simulink model "rx"  (R2019b)
settings: Solver=FixedStepDiscrete  StartTime=0.0  StopTime=inf  RelTol=1e-3
undefined symbols (not defined in the file): F, usb
libraries: plutoradiolib x1, commsink2 x1, zc706fmc234_lib x1
settings Model: Creator=tcollins  LastModifiedBy=bhisma
settings DataIOCC: ReturnWorkspaceOutputs=off
settings DebuggingCC: ArithmeticOperatorsInVariantConditions=warning
settings SFSimCC: SimUseLocalCustomCode=off  CustomCodeUndefinedFunction=UseInterfaceOnly
settings RTWCC: RTWUseLocalCustomCode=off

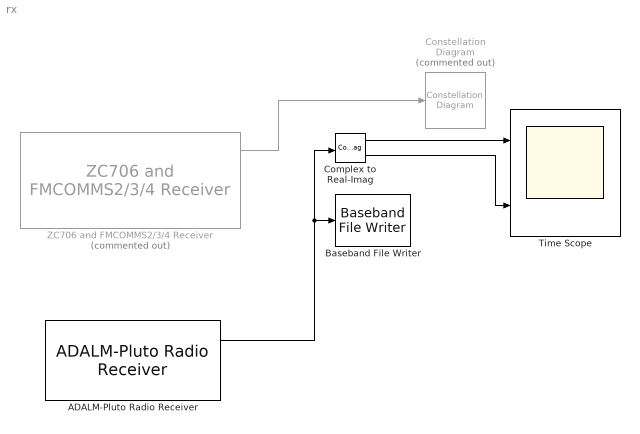
== system rx ==
  ADALM-Pluto Radio Receiver : plutoradiolib/ADALM-Pluto Radio Receiver  SourceLibraryInfo="This block requires <a href=\"http://www.mathworks.com/hardware-support/rtl-sdr.html\">Communications System Toolbox Support Package for RTL-SDR Radio</a>"  RadioID=usb:0  CenterFrequencySource=Dialog  CenterFrequency=2.4e9  GainSource=AGC Slow Attack  Gain=10  ChannelMapping=1  BasebandSampleRate=1e6  OutputDataType=int16  SamplesPerFrame=2^15  OverflowOutputPort=on  SimulateUsing=Interpreted execution  EnableQuadratureTracking=on  EnableRFDCTracking=on  EnableBasebandDCTracking=on
      settings: SourceProductName=Communications System Toolbox Support Package for ADALM-PLUTO Radio
  Baseband File Writer : commsink2/Baseband File Writer  Filename=untitled.bb  CenterFrequency=950e6  Metadata=struct()  NumSamplesToWrite=1e6  SimulateUsing=Code generation
      settings: SourceProductName=Communications Toolbox  SourceProductBaseCode=CM
  Complex to Real-Imag : ComplexToRealImag
  Constellation Diagram : ConstellationDiagram  Commented=on
  Time Scope : Scope  NumInputPorts=2
  ZC706 and FMCOMMS2/3/4 Receiver : zc706fmc234_lib/ZC706 and  FMCOMMS2//3//4  Receiver  Commented=on  IPAddress=192.168.3.2  CenterFrequencySource=Dialog  CenterFrequency=2.4e9  GainSource=AGC Slow Attack  Gain=1  ChannelMapping=1  BasebandSampleRate=20e6  EnableBurstMode=off  NumFramesInBurst=20  OutputDataType=int16  SamplesPerFrame=2^15  LostSamplesOutputPort=on  RSSIOutputPort=off  DMATimeoutValue=1  blockMode=Normal  SimulateUsing=Code generation  EnableQuadratureTracking=on  EnableRFDCTracking=on  EnableBasebandDCTracking=on  BypassUserLogic=on  ShowAdvancedProperties=on  ShowInternalProperties=off  subDeviceList=zynqReceiver  sdrExecutionMode=HW  dataUDPPort=-1  ctrlUDPPort=-1  SourceSelect=RF data  SourceConfiguration1=1023  FIRCoefficientSize=[128;128]  FIRCoefficients=[55 -54 42 -126 -123 -317 -399 -581 -646 -711 -634 -507 -263 -10 255 424 492 401 201 -84 -352 -540 -566 -423 -126 234 562 738 701 429 -5 -490 -866 -1007 -834 -372 266 891 1301 1334 936 178 -733 -1524 -1917 -1731 -944 274 1590 2585 2881 2255 741 -1344 -3435 -4850 -4942 -3285 197 5169 10923 16509 20932 23375 23375 20932 16509 10923 5169 197 -3285 -4942 -4850 -3435 -1344 741 2255 2881 2585 1590 274 -944 -1731 -1917 -1524 -733 178 936 1334 1301 891 266 -372 -834 -1007 -866 -490 -5 429 701 738 562 234 -126 -423 -566 -540 -352 -84 201 401 492 424 255 -10 -263 -507 -634 -711 -646 -581 -399 -317 -123 -126 42 -54 55;190 -88 329 -40 239 -99 -24 -349 -377 -611 -573 -604 -395 -229 66 239 394 350 227 -46 -300 -534 -593 -506 -221 137 512 737 765 526 103 -420 -852 -1069 -947 -512 156 841 1341 1450 1100 333 -638 -1531 -2028 -1922 -1152 115 1544 2677 3099 2535 997 -1205 -3479 -5095 -5345 -3750 -199 4965 11002 16895 21580 24172 24172 21580 16895 11002 4965 -199 -3750 -5345 -5095 -3479 -1205 997 2535 3099 2677 1544 115 -1152 -1922 -2028 -1531 -638 333 1100 1450 1341 841 156 -512 -947 -1069 -852 -420 103 526 765 737 512 137 -221 -506 -593 -534 -300 -46 227 350 394 239 66 -229 -395 -604 -573 -611 -377 -349 -24 -99 239 -40 329 -88 190]  FIRGain=[0;-12]  FIRDecimInterpFactor=[4;4]  AnalogFilterCutoff=[3152524;3161715]  FilterPathRates=[983040000 122880000 61440000 30720000 15360000 3840000;983040000 122880000 61440000 30720000 15360000 3840000]  FilterDesignTypeForTx=DefaultFilterFromOther  FilterDesignTypeForRx=DefaultFilter  BISTLoopbackConfig=No Loopback  BISTPRBSMode=PRBS Disable  BISTToneMode=Tone Disable  BISTToneFrequency=F/32  BISTToneLevel=-6  BISTChannelMask=0  DataIsComplex=on
      settings: SourceProductName=Communications Toolbox Support Package for Xilinx Zynq-Based Radio  SourceProductBaseCode=XILINXZYNQ
  wires:
  ZC706 and FMCOMMS2/3/4 Receiver/1 -> Constellation Diagram/1
  Complex to Real-Imag/1 -> Time Scope/1
  Complex to Real-Imag/2 -> Time Scope/2
  ADALM-Pluto Radio Receiver/1 -> Baseband File Writer/1, Complex to Real-Imag/1
